simulink model "CalculateTorqueLimits"  (R2026a)
settings: Solver=FixedStepDiscrete
model workspace (MAT data in the model file):
  Polepairs = Simulink.Parameter
  Polepairs.Value = 4
  Polepairs.Complexity = 'real'
  Polepairs.Dimensions = [1 1]
  Polepairs.DataType = 'auto'
settings Model: DataDictionary=TractionEmotorSoftwareArchInterfaceData.sldd  Creator=dakaihu  LastModifiedBy=dakaihu
settings OptimizationCC: GainParamInheritBuiltInType=on  UseFloatMulNetSlope=on  InlineInvariantSignals=on  NoFixptDivByZeroProtection=on  EfficientFloat2IntCast=on  LifeSpan=1
settings HardwareCC: ProdBitPerChar=16.0  ProdBitPerInt=16.0  ProdLargestAtomicInteger=Integer  ProdWordSize=16.0  ProdHWDeviceType=Texas Instruments->C2000
settings RTWCC: SystemTargetFile=ert.tlc  Description=Embedded Coder
settings CodeAppCC: MaxIdLength=60.0  CustomSymbolStrGlobalVar=rt$N$M  CustomSymbolStrType=$N$M  CustomSymbolStrFcn=$N$M$F  CustomSymbolStrMacro=$N$M
settings ERTTargetCC: ERTFilePackagingFormat=CompactWithDataFile  GenerateSampleERTMain=on  IncludeMdlTerminateFcn=off  CombineSignalStateStructs=on  SuppressErrorStatus=on  SupportAbsoluteTime=off  SupportComplex=off

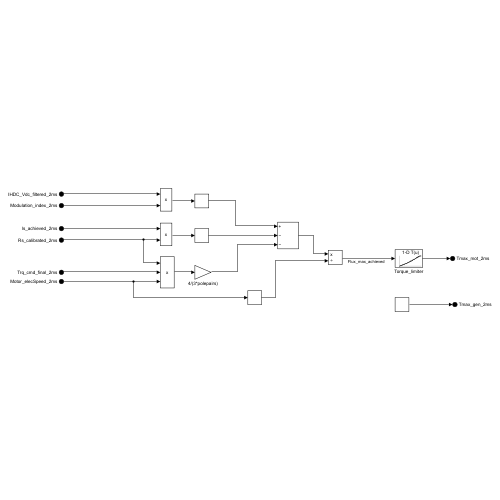
[thumbnail: Simulink's stored preview of the top-level diagram]
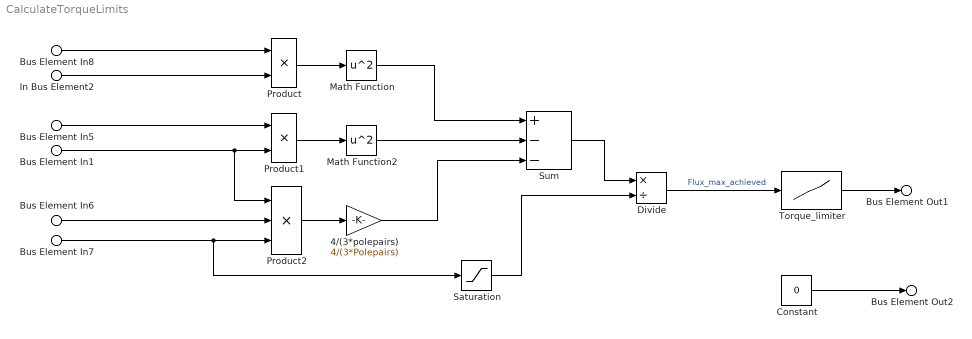
== system CalculateTorqueLimits ==
  Bus Element In5 : Inport  PortName=Is_achieved_2ms
  Bus Element In1 : Inport  Port=2  PortName=Rs_calibrated_2ms
  Bus Element In6 : Inport  Port=3  PortName=Trq_cmd_final_2ms
  Bus Element In7 : Inport  Port=4  PortName=Motor_elecSpeed_2ms
  Bus Element In8 : Inport  Port=5  PortName=IHDC_Vdc_filtered_2ms
  In Bus Element2 : Inport  Port=6  PortName=Modulation_index_2ms
  4/(3*polepairs) : Gain  Gain=4/(3*Polepairs)
  Constant : Constant  Value=0  SampleTime=-1
  Divide : Product  Inputs=*/
  Math Function : Math  Operator=square
  Math Function2 : Math  Operator=square
  Product : Product
  Product1 : Product
  Product2 : Product  Inputs=3
  Saturation : Saturate  UpperLimit=inf  LowerLimit=0.1
  Sum : Sum  Inputs=+--
  Torque_limiter : Lookup_n-D  NumberOfTableDimensions=1  BreakpointsForDimension1=|  Table=|  ExtrapMethod=Clip  UseLastTableValue=on  InternalRulePriority=Speed  RndMeth=Simplest
      BreakpointsForDimension1=|
      | [0.0892746623589603383
      | 0.0971549350626077779
      | 0.104193581417730718
      | 0.111166676863611105
      | 0.118066366738619172
      | 0.124887196094081318
      | 0.131657648447774139
      | 0.138388024625694883
      | 0.145072733636910339
      | 0.15170471535466426
      | 0.158277815768927022
      | 0.164787137330455302
      | 0.171228069598704263
      | 0.177597658195089991
      | 0.183891217638001175
      | 0.190099150416764701
      | 0.196212479661762057
      | 0.202227064904261733
      | 0.208138992678437829
      | 0.213944671773418055
      | 0.219641390694035571
      | 0.225231075673947317
      | 0.230744605954803395
      | 0.236200922970522087
      | 0.241602698906775354
      | 0.246951788950300094
      | 0.252247068388392115
      | 0.257485670105000619
      | 0.262662971699388126
      | 0.26777369460094097
      | 0.272811495936155557
      | 0.277767284979567264
      | 0.282633824418224266
      | 0.287402395173474379
      | 0.292060818394260513
      | 0.296601956882838025
      | 0.301022778863190565
      | 0.305325166633790113
      | 0.309517828659907013
      | 0.313603456336929542
      | 0.317581041938773068
      | 0.321449156446341366
      | 0.325215790040922492
      | 0.328881705248184386
      | 0.332452423767418681
      | 0.335930280117159252
      | 0.339314002381673085
      | 0.34260829849660257
      | 0.345813654935997861
      | 0.348911398091495351
      | 0.34969684430679665
      | 0.35192795416605771
      | 0.354074970516559839
      | 0.356141250993826819
      | 0.358133752536437866
      | 0.360056687764013672
      | 0.361917557294053727
      | 0.363720358060084958
      | 0.365473585655795796
      | 0.367178803898214556
      | 0.368848396550364777
      | 0.370485065272030789
      | 0.372098744067622278
      | 0.373693320895818692
      | 0.375262797987825969
      | 0.37677922281905929
      | 0.378237897356784591
      | 0.379646385428738853
      | 0.381006632433825654
      | 0.382322927140264224
      | 0.383600818421808931
      | 0.384841119074542104
      | 0.38604989726768979
      | 0.387231341900532433
      | 0.388385709805056933
      | 0.389519436509782768
      | 0.390635965594523793
      | 0.391735076708492502
      | 0.392823020446009974
      | 0.393898376884281365
      | 0.39494385868749815
      | 0.395957713891687657
      | 0.396942408464295182
      | 0.397899656095757892
      | 0.398829090926657248
      | 0.399734072872468871
      | 0.401423102353018535]
      Table=|
      | [71.0563209760550052
      | 77.8998952548809029
      | 84.1161466370865014
      | 90.3815783939901962
      | 96.6949346188427938
      | 103.055362287641003
      | 109.492016194561003
      | 116.023490768849001
      | 122.640237659576997
      | 129.331853846401998
      | 136.087449859668993
      | 142.896595288243986
      | 149.74814900828099
      | 156.631080482273006
      | 163.536814146947989
      | 170.451048668445992
      | 177.35864257979901
      | 184.247034707963991
      | 191.104113087868996
      | 197.917410224306991
      | 204.675313675339993
      | 211.374478822420002
      | 218.070909554545011
      | 224.79144321880301
      | 231.536119187657988
      | 238.301678609548986
      | 245.080830482268993
      | 251.862331048549009
      | 258.633817812242
      | 265.382062727527
      | 272.092951169913988
      | 278.751164622553972
      | 285.341119153596026
      | 291.842961303894981
      | 298.242689391906026
      | 304.52508346825698
      | 310.693427648089028
      | 316.769125652738978
      | 322.751411321995988
      | 328.641779304679005
      | 334.443411128816024
      | 340.163120321138024
      | 345.802516864153972
      | 351.36199457626202
      | 356.832067215898007
      | 362.217455040437983
      | 367.514276985811023
      | 372.713309140159993
      | 377.800580249841005
      | 382.765835847444976
      | 384.008346109405977
      | 387.464040878388005
      | 390.709617962261007
      | 393.757605901301019
      | 396.619451666978023
      | 399.307018600320021
      | 401.836853504046019
      | 404.221601942307018
      | 406.473828088928997
      | 408.60613691074002
      | 410.631092695716006
      | 412.561267414546023
      | 414.409184759242976
      | 416.187283353876012
      | 417.886909351825977
      | 419.457841990478016
      | 420.902815126827022
      | 422.23068676654799
      | 423.449921586132007
      | 424.568605399482976
      | 425.594276021808014
      | 426.534353627895996
      | 427.395737099171015
      | 428.184742266324008
      | 428.907494941529023
      | 429.569794741329986
      | 430.176634660666025
      | 430.733116145619988
      | 431.243870464894997
      | 431.707559716639025
      | 432.103052797147996
      | 432.427479224152023
      | 432.682504373056986
      | 432.87212580137998
      | 432.99994926177402
      | 433.068829467128978
      | 433.044752905119992]
  Bus Element Out1 : Outport  PortName=Tmax_mot_2ms
  Bus Element Out2 : Outport  Port=2  PortName=Tmax_gen_2ms
  wires:
  Bus Element In5/1 -> Product1/1
  Product/1 -> Math Function/1
  Bus Element In1/1 -> Product2/1, Product1/2
  Divide/1 -> Torque_limiter/1  "Flux_max_achieved"
  Math Function2/1 -> Sum/2
  4/(3*polepairs)/1 -> Sum/3
  In Bus Element2/1 -> Product/2
  Bus Element In6/1 -> Product2/2
  Math Function/1 -> Sum/1
  Bus Element In8/1 -> Product/1
  Product2/1 -> 4/(3*polepairs)/1
  Bus Element In7/1 -> Saturation/1, Product2/3
  Sum/1 -> Divide/1
  Product1/1 -> Math Function2/1
  Torque_limiter/1 -> Bus Element Out1/1
  Constant/1 -> Bus Element Out2/1
  Saturation/1 -> Divide/2
